simulink model "Lab1_Model4"  (R2021b)
settings: Solver=FixedStepDiscrete  StartTime=0.0  StopTime=10  FixedStep=T  RelTol=1e-3  EnableMultiTasking=on
libraries: cstblocks x2
settings Model: Creator=sarth  LastModifiedBy=sarth

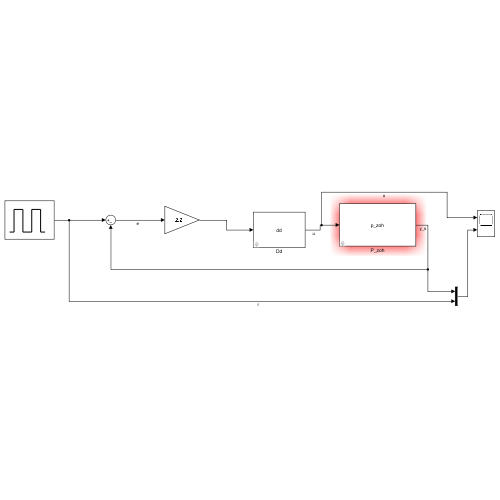
[thumbnail: Simulink's stored preview of the top-level diagram]
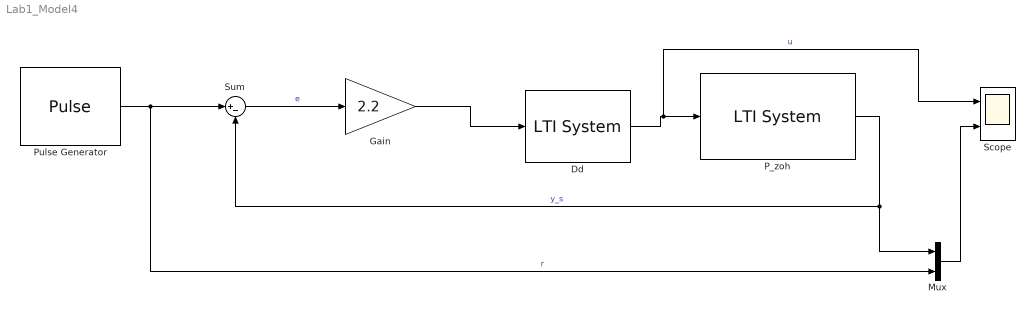
== system Lab1_Model4 ==
  Dd : cstblocks/LTI System  sys=dd  IC=[]
  Gain : Gain  Gain=2.2
  Mux : Mux  Inputs=2
  P_zoh : cstblocks/LTI System  sys=p_zoh  IC=[]
  Pulse Generator : DiscretePulseGenerator  PulseType=Time based  Period=10  PulseWidth=50
  Scope : Scope  NumInputPorts=2
  Sum : Sum  Inputs=|+-
  wires:
  Pulse Generator/1 -> Mux/2, Sum/1  "r"
  Mux/1 -> Scope/2
  Sum/1 -> Gain/1  "e"
  P_zoh/1 -> Sum/2, Mux/1  "y_s"
  Gain/1 -> Dd/1
  Dd/1 -> Scope/1, P_zoh/1  "u"
